simulink model "GD_Termoeletrica_Isolada_Droop"  (R2025b)
settings: Solver=ode23t  StartTime=0.0  StopTime=10  RelTol=1e-3  EnableMultiTasking=on
undefined symbols (not defined in the file): Three_PhaseV_IMeasuremen_class
libraries: fl_lib x9, nesl_utility x9, ee_lib x6, slpidlib x2, sdl_lib x2, AvgModels x1
settings Model: Creator=lgalo
settings SolverCC: AlgebraicLoopSolver=TrustRegion
settings DataIOCC: LimitDataPoints=on  SaveFormat=Array  ReturnWorkspaceOutputs=off
settings OptimizationCC: LifeSpan=inf
settings DebuggingCC: SaveWithParameterizedLinksMsg=none  UnconnectedInputMsg=warning  UnconnectedOutputMsg=warning  UnconnectedLineMsg=warning  SFUnexpectedBacktrackingDiag=warning  SFNoUnconditionalDefaultTransitionDiag=warning  SFExecutionAtInitializationDiag=none  ArithmeticOperatorsInVariantConditions=warning
settings HardwareCC: ProdBitPerPointer=32.0  ProdBitPerSizeT=32.0  ProdBitPerPtrDiffT=32.0  ProdLargestAtomicFloat=None  ProdIntDivRoundTo=Undefined  ProdEndianess=Unspecified  ProdWordSize=32.0  ProdHWDeviceType=32-bit Generic
settings ModelReferenceCC: PropagateSignalLabelsOutOfModel=off
settings SFSimCC: SimUseLocalCustomCode=off  CustomCodeUndefinedFunction=UseInterfaceOnly
settings RTWCC: RTWUseLocalCustomCode=off  GPUComputeCapability=3.5
settings CodeAppCC: StateflowObjectComments=on
settings GRTTargetCC: TargetLangStandard=C89/C90 (ANSI)
settings ConfigComp: CovMetricSettings=dw  CovSaveCumulativeToWorkspaceVar=on  CovSaveSingleToWorkspaceVar=on  CovExternalEMLEnable=off
settings SimscapeCC: SimscapeNormalizeSystem=off

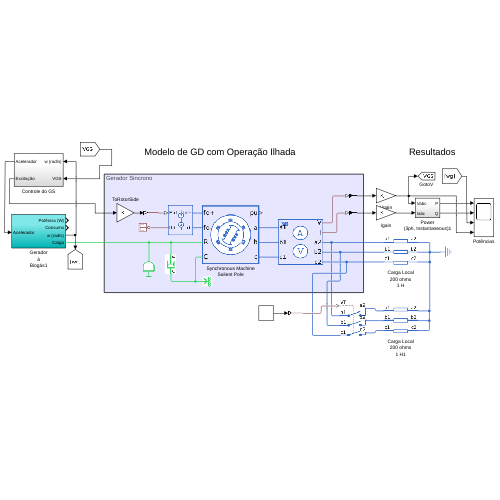
[thumbnail: Simulink's stored preview of the top-level diagram]
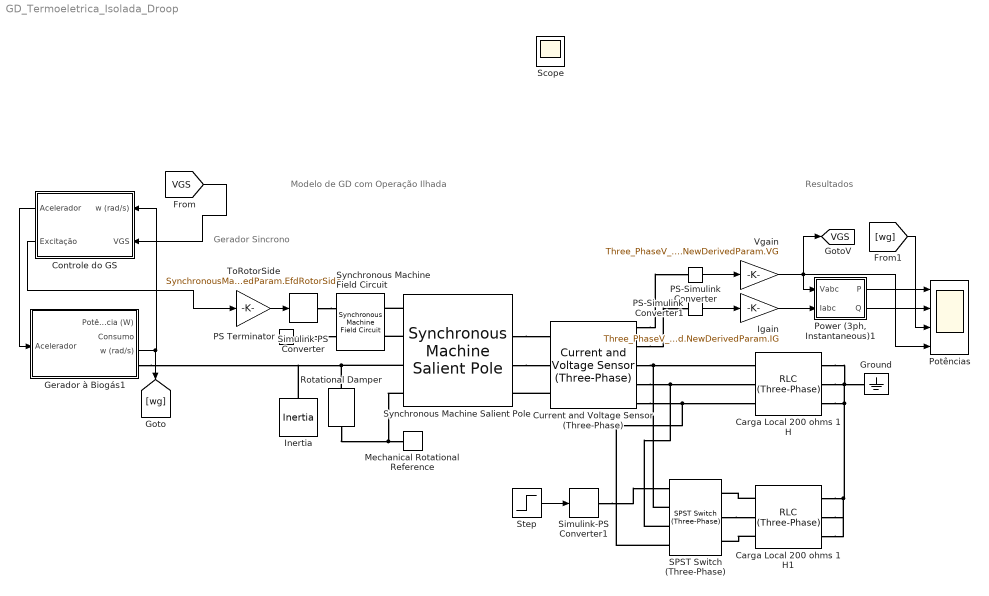
== system GD_Termoeletrica_Isolada_Droop ==
  note: Gerador Sincrono
  note: Modelo de GD com Operação Ilhada
  note: Resultados
  Carga Local 200 ohms 1 H : ee_lib/Passive/RLC Assemblies/RLC (Three-Phase)  port_option=ee.enum.threePhasePort.expanded  component_structure=8  R=200 Ohm  L=1 H  C=1e-06 F  R_parasitic=1e-6 Ohm  G_parasitic=1e-6 1/Ohm  IL_specify=on  IL_priority=High  IL=[0, 0, 0] A  IL_nominal_specify=off  IL_nominal_value=1  IL_nominal_unit=A  VC_specify=on  VC_priority=High  VC=[0, 0, 0] V  VC_nominal_specify=off  VC_nominal_value=1  VC_nominal_unit=V
      settings: InternalSimscapePortConfiguration="{\"Bottom\":[],\"Left\":[{\"id\":\"a1\",\"label\":\"a1\",\"type\":\"foundation.electrical.electrical\"},{\"id\":\"b1\",\"label\":\"b1\",\"type\":\"foundation.electrical.electrical\"},{\"id\":\"c1\",\"label\":\"c1\",\"type\":\"foundation.electrical.electrical\"}],\"Right\":[{\"id\":\"a2\",\"label\":\"a2\",\"type\":\"foundation.electrical.electrical\"},{\"id\":\"b2\",\"label\":\"b2\",\"type\":\"foundation.electrical.electrical\"},{\"id\":\"c2\",\"label\":\"c2\",\"type\":\"foundation.electrical.electrical\"}],\"Top\":[]}"
  Carga Local 200 ohms 1 H1 : ee_lib/Passive/RLC Assemblies/RLC (Three-Phase)  port_option=ee.enum.threePhasePort.expanded  component_structure=8  R=200 Ohm  L=1 H  C=1e-06 F  R_parasitic=1e-6 Ohm  G_parasitic=1e-6 1/Ohm  IL_specify=on  IL_priority=High  IL=[0, 0, 0] A  IL_nominal_specify=off  IL_nominal_value=1  IL_nominal_unit=A  VC_specify=on  VC_priority=High  VC=[0, 0, 0] V  VC_nominal_specify=off  VC_nominal_value=1  VC_nominal_unit=V
      settings: InternalSimscapePortConfiguration="{\"Bottom\":[],\"Left\":[{\"id\":\"a1\",\"label\":\"a1\",\"type\":\"foundation.electrical.electrical\"},{\"id\":\"b1\",\"label\":\"b1\",\"type\":\"foundation.electrical.electrical\"},{\"id\":\"c1\",\"label\":\"c1\",\"type\":\"foundation.electrical.electrical\"}],\"Right\":[{\"id\":\"a2\",\"label\":\"a2\",\"type\":\"foundation.electrical.electrical\"},{\"id\":\"b2\",\"label\":\"b2\",\"type\":\"foundation.electrical.electrical\"},{\"id\":\"c2\",\"label\":\"c2\",\"type\":\"foundation.electrical.electrical\"}],\"Top\":[]}"
  Controle do GS : Subsystem
  Current and Voltage Sensor (Three-Phase) : ee_lib/Sensors & Transducers/Current and Voltage Sensor (Three-Phase)  vMeasurementType=2  outputUnit=2  SRated=100000000 V*A  VRated=500000 V  I_specify=off  I_priority=None  I=[ 0 0 0 ] A  I_nominal_specify=off  I_nominal_value=1  I_nominal_unit=A  V_specify=off  V_priority=None  V=[ 0 0 0 ] V  V_nominal_specify=off  V_nominal_value=1  V_nominal_unit=V
      settings: InternalSimscapePortConfiguration="{\"Bottom\":[],\"Left\":[{\"id\":\"a1\",\"label\":\"a1\",\"type\":\"foundation.electrical.electrical\"},{\"id\":\"b1\",\"label\":\"b1\",\"type\":\"foundation.electrical.electrical\"},{\"id\":\"c1\",\"label\":\"c1\",\"type\":\"foundation.electrical.electrical\"}],\"Right\":[{\"id\":\"V_output\",\"label\":\"V\",\"type\":\"output\"},{\"id\":\"I_output\",\"label\":\"I\",\"type\":\"output\"},{\"id\":\"a2\",\"label\":\"a2\",\"type\":\"foundation.electrical.electrical\"},{\"id\":\"b2\",\"label\":\"b2\",\"type\":\"foundation.electrical.electrical\"},{\"id\":\"c2\",\"label\":\"c2\",\"type\":\"foundation.electrical.electrical\"}],\"Top\":[]}"
  Gerador à Biogás1 : Subsystem
  Ground : fl_lib/Electrical/Electrical Elements/Electrical Reference
  Igain : Gain  Gain=Three_PhaseV_IMeasuremen_class('phase-to-ground','yes','off','off','off',100000000,500000).objParamMappingDerived.NewDerivedParam.IG
  Inertia : fl_lib/Mechanical/Rotational Elements/Inertia  inertia=SynchronousMachineSIFund_class('Mechanical rotational port',[20000 460 60],[0.645 0.002217 0.05296 0.0252],[0.1279 0.016 2],2,[0 0 0 0 0 0 0 0 1.3192],[695.64 774.7 917.5 1001.6 1082.2 1175.9 1293.6 1430.2 1583.7;9660 10623 12243 13063 13757 14437 15180 15890 16567],'off',[0.0664 0.001387 0.0292 0.0006896 0.007907 0.002477],[1.137 0.00419 1.54 0.004893],[0.3802 0.005517],'Salient-pole').objParamMappingDerived.NewDerivedParam.J kg*m^2  num_ports=foundation.enum.numPorts2.one  w_specify=on  w_priority=Low  w=SynchronousMachineSIFund_class('Mechanical rotational port',[20000 460 60],[0.645 0.002217 0.05296 0.0252],[0.1279 0.016 2],2,[0 0 0 0 0 0 0 0 1.3192],[695.64 774.7 917.5 1001.6 1082.2 1175.9 1293.6 1430.2 1583.7;9660 10623 12243 13063 13757 14437 15180 15890 16567],'off',[0.0664 0.001387 0.0292 0.0006896 0.007907 0.002477],[1.137 0.00419 1.54 0.004893],[0.3802 0.005517],'Salient-pole').objParamMappingDerived.NewDerivedParam.wrm0 rad/s  w_nominal_specify=off  w_nominal_value=1  w_nominal_unit=rad/s  t_specify=off  t_priority=None  t=0 N*m  t_nominal_specify=off  t_nominal_value=1  t_nominal_unit=N*m
  Mechanical Rotational Reference : fl_lib/Mechanical/Rotational Elements/Mechanical Rotational Reference
  PS Terminator : fl_lib/Physical Signals/Sinks/PS Terminator
  PS-Simulink Converter : nesl_utility/PS-Simulink Converter  PhysicalDomain=network_engine_domain  SubClassName=ps_output  LeftPortType=input  RightPortType=output  PseudoPeriodic=off  Frequencies=[]  VectorFormat=1-D array  Unit=1  AffineConversion=off
  PS-Simulink Converter1 : nesl_utility/PS-Simulink Converter  PhysicalDomain=network_engine_domain  SubClassName=ps_output  LeftPortType=input  RightPortType=output  PseudoPeriodic=off  Frequencies=[]  VectorFormat=1-D array  Unit=1  AffineConversion=off
  Potências : Scope  NumInputPorts=4
      settings: TimeSpan=10  ActiveDisplayYMinimum=-98.69848861877999  ActiveDisplayYMaximum=888.28639756902021  DataLoggingSaveFormat=Array
  "Power (3ph, Instantaneous)1" : Subsystem
  Rotational Damper : fl_lib/Mechanical/Rotational Elements/Rotational Damper  D=SynchronousMachineSIFund_class('Mechanical rotational port',[20000 460 60],[0.645 0.002217 0.05296 0.0252],[0.1279 0.016 2],2,[0 0 0 0 0 0 0 0 1.3192],[695.64 774.7 917.5 1001.6 1082.2 1175.9 1293.6 1430.2 1583.7;9660 10623 12243 13063 13757 14437 15180 15890 16567],'off',[0.0664 0.001387 0.0292 0.0006896 0.007907 0.002477],[1.137 0.00419 1.54 0.004893],[0.3802 0.005517],'Salient-pole').objParamMappingDerived.NewDerivedParam.D N*m/(rad/s)  w_specify=on  w_priority=Low  w=SynchronousMachineSIFund_class('Mechanical rotational port',[20000 460 60],[0.645 0.002217 0.05296 0.0252],[0.1279 0.016 2],2,[0 0 0 0 0 0 0 0 1.3192],[695.64 774.7 917.5 1001.6 1082.2 1175.9 1293.6 1430.2 1583.7;9660 10623 12243 13063 13757 14437 15180 15890 16567],'off',[0.0664 0.001387 0.0292 0.0006896 0.007907 0.002477],[1.137 0.00419 1.54 0.004893],[0.3802 0.005517],'Salient-pole').objParamMappingDerived.NewDerivedParam.wrm0 rad/s  w_nominal_specify=off  w_nominal_value=1  w_nominal_unit=rad/s  t_specify=off  t_priority=None  t=0 N*m  t_nominal_specify=off  t_nominal_value=1  t_nominal_unit=N*m
  SPST Switch (Three-Phase) : ee_lib/Switches & Breakers/SPST Switch (Three-Phase)  R_closed=0.001 Ohm  G_open=1e-6 1/Ohm  threshold=0.5 V  i_vT_specify=off  i_vT_priority=None  i_vT=0 A  i_vT_nominal_specify=off  i_vT_nominal_value=1  i_vT_nominal_unit=A  I_specify=off  I_priority=None  I=[0, 0, 0] A  I_nominal_specify=off  I_nominal_value=1  I_nominal_unit=A  V_specify=off  V_priority=None  V=[0, 0, 0] V  V_nominal_specify=off  V_nominal_value=1  V_nominal_unit=V  i_a_specify=off  i_a_priority=None  i_a=0 A  i_a_nominal_specify=off  i_a_nominal_value=1  i_a_nominal_unit=A  v_a_specify=off  v_a_priority=None  v_a=0 V  v_a_nominal_specify=off  v_a_nominal_value=1  v_a_nominal_unit=V  i_b_specify=off  i_b_priority=None  i_b=0 A  i_b_nominal_specify=off  i_b_nominal_value=1  i_b_nominal_unit=A  v_b_specify=off  v_b_priority=None  v_b=0 V  v_b_nominal_specify=off  v_b_nominal_value=1  v_b_nominal_unit=V  i_c_specify=off  i_c_priority=None  i_c=0 A  i_c_nominal_specify=off  i_c_nominal_value=1  i_c_nominal_unit=A  v_c_specify=off  v_c_priority=None  v_c=0 V  v_c_nominal_specify=off  v_c_nominal_value=1  v_c_nominal_unit=V
      settings: InternalSimscapePortConfiguration="{\"Bottom\":[],\"Left\":[{\"id\":\"vT\",\"label\":\"vT\",\"type\":\"input\"},{\"id\":\"a1\",\"label\":\"a1\",\"type\":\"foundation.electrical.electrical\"},{\"id\":\"b1\",\"label\":\"b1\",\"type\":\"foundation.electrical.electrical\"},{\"id\":\"c1\",\"label\":\"c1\",\"type\":\"foundation.electrical.electrical\"}],\"Right\":[{\"id\":\"a2\",\"label\":\"a2\",\"type\":\"foundation.electrical.electrical\"},{\"id\":\"b2\",\"label\":\"b2\",\"type\":\"foundation.electrical.electrical\"},{\"id\":\"c2\",\"label\":\"c2\",\"type\":\"foundation.electrical.electrical\"}],\"Top\":[]}"
  Simulink-PS Converter : nesl_utility/Simulink-PS Converter  PhysicalDomain=network_engine_domain  SubClassName=ps_input  LeftPortType=input  RightPortType=output  PseudoPeriodic=off  Frequencies=[]  NoiseDistribution=none  NoiseParameters=[]  Unit=1  AffineConversion=off  FilteringAndDerivatives=provide  SimscapeFilterOrder=1  InputFilterTimeConstant=0.001  UdotUserProvided=0
  Simulink-PS Converter1 : nesl_utility/Simulink-PS Converter  PhysicalDomain=network_engine_domain  SubClassName=ps_input  LeftPortType=input  RightPortType=output  PseudoPeriodic=off  Frequencies=[]  NoiseDistribution=none  NoiseParameters=[]  Unit=1  AffineConversion=off  FilteringAndDerivatives=provide  SimscapeFilterOrder=1  InputFilterTimeConstant=0.001  UdotUserProvided=0
  Step : Step  Time=5  SampleTime=0
  Synchronous Machine Field Circuit : ee_lib/Electromechanical/Synchronous/Synchronous Machine Field Circuit  unit_option=ee.enum.unit.si  SRated=555e6 V*A  FRated=60 Hz  fieldCircuitParameterization_option=ee.enum.sm.fieldparameterization.current  baseEfd=92.95 V  baseIfd=1300 A  parameterization_option=ee.enum.sm.parameterization.fundamental  Ladu=1.66  Rfd=0.0006  Xl=0.15  Xd=1.81  Xdd=0.3  Xddd=0.23  d_option=ee.enum.circuit.open  Td0d=8 s  Tdd=1.3260 s  Td0dd=0.03 s  Tddd=0.0230 s
      settings: InternalSimscapePortConfiguration="{\"Bottom\":[],\"Left\":[{\"id\":\"Efd\",\"label\":\"Efd\",\"type\":\"input\"},{\"id\":\"Ifd\",\"label\":\"Ifd\",\"type\":\"output\"}],\"Right\":[{\"id\":\"fd_p\",\"label\":\"fd+\",\"type\":\"foundation.electrical.electrical\"},{\"id\":\"fd_n\",\"label\":\"fd-\",\"type\":\"foundation.electrical.electrical\"}],\"Top\":[]}"
  Synchronous Machine Salient Pole : ee_lib/Electromechanical/Synchronous/Synchronous Machine Salient Pole  port_option=ee.enum.threePhasePort.expanded  SRated=SynchronousMachineSIFund_class('Mechanical rotational port',[20000 460 60],[0.645 0.002217 0.05296 0.0252],[0.1279 0.016 2],2,[0 0 0 0 0 0 0 0 1.3192],[695.64 774.7 917.5 1001.6 1082.2 1175.9 1293.6 1430.2 1583.7;9660 10623 12243 13063 13757 14437 15180 15890 16567],'off',[0.0664 0.001387 0.0292 0.0006896 0.007907 0.002477],[1.137 0.00419 1.54 0.004893],[0.3802 0.005517],'Salient-pole').objParamMappingDerived.NewDerivedParam.SRated V*A  VRated=SynchronousMachineSIFund_class('Mechanical rotational port',[20000 460 60],[0.645 0.002217 0.05296 0.0252],[0.1279 0.016 2],2,[0 0 0 0 0 0 0 0 1.3192],[695.64 774.7 917.5 1001.6 1082.2 1175.9 1293.6 1430.2 1583.7;9660 10623 12243 13063 13757 14437 15180 15890 16567],'off',[0.0664 0.001387 0.0292 0.0006896 0.007907 0.002477],[1.137 0.00419 1.54 0.004893],[0.3802 0.005517],'Salient-pole').objParamMappingDerived.NewDerivedParam.VRated V  FRated=SynchronousMachineSIFund_class('Mechanical rotational port',[20000 460 60],[0.645 0.002217 0.05296 0.0252],[0.1279 0.016 2],2,[0 0 0 0 0 0 0 0 1.3192],[695.64 774.7 917.5 1001.6 1082.2 1175.9 1293.6 1430.2 1583.7;9660 10623 12243 13063 13757 14437 15180 15890 16567],'off',[0.0664 0.001387 0.0292 0.0006896 0.007907 0.002477],[1.137 0.00419 1.54 0.004893],[0.3802 0.005517],'Salient-pole').objParamMappingDerived.NewDerivedParam.FRated Hz  nPolePairs=SynchronousMachineSIFund_class('Mechanical rotational port',[20000 460 60],[0.645 0.002217 0.05296 0.0252],[0.1279 0.016 2],2,[0 0 0 0 0 0 0 0 1.3192],[695.64 774.7 917.5 1001.6 1082.2 1175.9 1293.6 1430.2 1583.7;9660 10623 12243 13063 13757 14437 15180 15890 16567],'off',[0.0664 0.001387 0.0292 0.0006896 0.007907 0.002477],[1.137 0.00419 1.54 0.004893],[0.3802 0.005517],'Salient-pole').objParamMappingDerived.NewDerivedParam.nPolePairs  param_option=ee.enum.sm.parameterization.fundamental  fieldCircuitParameterization_option=ee.enum.sm.fieldparameterization.current  baseEfd=216.54 V  baseIfd=SynchronousMachineSIFund_class('Mechanical rotational port',[20000 460 60],[0.645 0.002217 0.05296 0.0252],[0.1279 0.016 2],2,[0 0 0 0 0 0 0 0 1.3192],[695.64 774.7 917.5 1001.6 1082.2 1175.9 1293.6 1430.2 1583.7;9660 10623 12243 13063 13757 14437 15180 15890 16567],'off',[0.0664 0.001387 0.0292 0.0006896 0.007907 0.002477],[1.137 0.00419 1.54 0.004893],[0.3802 0.005517],'Salient-pole').objParamMappingDerived.NewDerivedParam.baseIfd A  zero_sequence=ee.enum.park.zerosequence.exclude  axes_param=ee.enum.rotorangle.qaxis  Ladu=SynchronousMachineSIFund_class('Mechanical rotational port',[20000 460 60],[0.645 0.002217 0.05296 0.0252],[0.1279 0.016 2],2,[0 0 0 0 0 0 0 0 1.3192],[695.64 774.7 917.5 1001.6 1082.2 1175.9 1293.6 1430.2 1583.7;9660 10623 12243 13063 13757 14437 15180 15890 16567],'off',[0.0664 0.001387 0.0292 0.0006896 0.007907 0.002477],[1.137 0.00419 1.54 0.004893],[0.3802 0.005517],'Salient-pole').objParamMappingDerived.NewDerivedParam.Ladu  Laqu=SynchronousMachineSIFund_class('Mechanical rotational port',[20000 460 60],[0.645 0.002217 0.05296 0.0252],[0.1279 0.016 2],2,[0 0 0 0 0 0 0 0 1.3192],[695.64 774.7 917.5 1001.6 1082.2 1175.9 1293.6 1430.2 1583.7;9660 10623 12243 13063 13757 14437 15180 15890 16567],'off',[0.0664 0.001387 0.0292 0.0006896 0.007907 0.002477],[1.137 0.00419 1.54 0.004893],[0.3802 0.005517],'Salient-pole').objParamMappingDerived.NewDerivedParam.Laqu  L0=SynchronousMachineSIFund_class('Mechanical rotational port',[20000 460 60],[0.645 0.002217 0.05296 0.0252],[0.1279 0.016 2],2,[0 0 0 0 0 0 0 0 1.3192],[695.64 774.7 917.5 1001.6 1082.2 1175.9 1293.6 1430.2 1583.7;9660 10623 12243 13063 13757 14437 15180 15890 16567],'off',[0.0664 0.001387 0.0292 0.0006896 0.007907 0.002477],[1.137 0.00419 1.54 0.004893],[0.3802 0.005517],'Salient-pole').objParamMappingDerived.NewDerivedParam.L0  Ll=SynchronousMachineSIFund_class('Mechanical rotational port',[20000 460 60],[0.645 0.002217 0.05296 0.0252],[0.1279 0.016 2],2,[0 0 0 0 0 0 0 0 1.3192],[695.64 774.7 917.5 1001.6 1082.2 1175.9 1293.6 1430.2 1583.7;9660 10623 12243 13063 13757 14437 15180 15890 16567],'off',[0.0664 0.001387 0.0292 0.0006896 0.007907 0.002477],[1.137 0.00419 1.54 0.004893],[0.3802 0.005517],'Salient-pole').objParamMappingDerived.NewDerivedParam.Ll  Ra=SynchronousMachineSIFund_class('Mechanical rotational port',[20000 460 60],[0.645 0.002217 0.05296 0.0252],[0.1279 0.016 2],2,[0 0 0 0 0 0 0 0 1.3192],[695.64 774.7 917.5 1001.6 1082.2 1175.9 1293.6 1430.2 1583.7;9660 10623 12243 13063 13757 14437 15180 15890 16567],'off',[0.0664 0.001387 0.0292 0.0006896 0.007907 0.002477],[1.137 0.00419 1.54 0.004893],[0.3802 0.005517],'Salient-pole').objParamMappingDerived.NewDerivedParam.Ra  Lfd=SynchronousMachineSIFund_class('Mechanical rotational port',[20000 460 60],[0.645 0.002217 0.05296 0.0252],[0.1279 0.016 2],2,[0 0 0 0 0 0 0 0 1.3192],[695.64 774.7 917.5 1001.6 1082.2 1175.9 1293.6 1430.2 1583.7;9660 10623 12243 13063 13757 14437 15180 15890 16567],'off',[0.0664 0.001387 0.0292 0.0006896 0.007907 0.002477],[1.137 0.00419 1.54 0.004893],[0.3802 0.005517],'Salient-pole').objParamMappingDerived.NewDerivedParam.Lfd  Rfd=SynchronousMachineSIFund_class('Mechanical rotational port',[20000 460 60],[0.645 0.002217 0.05296 0.0252],[0.1279 0.016 2],2,[0 0 0 0 0 0 0 0 1.3192],[695.64 774.7 917.5 1001.6 1082.2 1175.9 1293.6 1430.2 1583.7;9660 10623 12243 13063 13757 14437 15180 15890 16567],'off',[0.0664 0.001387 0.0292 0.0006896 0.007907 0.002477],[1.137 0.00419 1.54 0.004893],[0.3802 0.005517],'Salient-pole').objParamMappingDerived.NewDerivedParam.Rfd  L1d=SynchronousMachineSIFund_class('Mechanical rotational port',[20000 460 60],[0.645 0.002217 0.05296 0.0252],[0.1279 0.016 2],2,[0 0 0 0 0 0 0 0 1.3192],[695.64 774.7 917.5 1001.6 1082.2 1175.9 1293.6 1430.2 1583.7;9660 10623 12243 13063 13757 14437 15180 15890 16567],'off',[0.0664 0.001387 0.0292 0.0006896 0.007907 0.002477],[1.137 0.00419 1.54 0.004893],[0.3802 0.005517],'Salient-pole').objParamMappingDerived.NewDerivedParam.L1d  R1d=SynchronousMachineSIFund_class('Mechanical rotational port',[20000 460 60],[0.645 0.002217 0.05296 0.0252],[0.1279 0.016 2],2,[0 0 0 0 0 0 0 0 1.3192],[695.64 774.7 917.5 1001.6 1082.2 1175.9 1293.6 1430.2 1583.7;9660 10623 12243 13063 13757 14437 15180 15890 16567],'off',[0.0664 0.001387 0.0292 0.0006896 0.007907 0.002477],[1.137 0.00419 1.54 0.004893],[0.3802 0.005517],'Salient-pole').objParamMappingDerived.NewDerivedParam.R1d  L1q=SynchronousMachineSIFund_class('Mechanical rotational port',[20000 460 60],[0.645 0.002217 0.05296 0.0252],[0.1279 0.016 2],2,[0 0 0 0 0 0 0 0 1.3192],[695.64 774.7 917.5 1001.6 1082.2 1175.9 1293.6 1430.2 1583.7;9660 10623 12243 13063 13757 14437 15180 15890 16567],'off',[0.0664 0.001387 0.0292 0.0006896 0.007907 0.002477],[1.137 0.00419 1.54 0.004893],[0.3802 0.005517],'Salient-pole').objParamMappingDerived.NewDerivedParam.L1q  R1q=SynchronousMachineSIFund_class('Mechanical rotational port',[20000 460 60],[0.645 0.002217 0.05296 0.0252],[0.1279 0.016 2],2,[0 0 0 0 0 0 0 0 1.3192],[695.64 774.7 917.5 1001.6 1082.2 1175.9 1293.6 1430.2 1583.7;9660 10623 12243 13063 13757 14437 15180 15890 16567],'off',[0.0664 0.001387 0.0292 0.0006896 0.007907 0.002477],[1.137 0.00419 1.54 0.004893],[0.3802 0.005517],'Salient-pole').objParamMappingDerived.NewDerivedParam.R1q  Xl=0.15  Xd=1.05  Xq=0.7  X0=0.15  Xdd=0.35  Xddd=0.25  Xqdd=0.325  d_option=ee.enum.circuit.open  Td0d=5.25 s  Tdd=1.75 s  Td0dd=0.03 s  Tddd=0.0214 s  q_option=ee.enum.circuit.open  Tq0dd=0.05 s  Tqdd=0.0232 s  saturation_option=0  saturation_ifd=SynchronousMachineSIFund_class('Mechanical rotational port',[20000 460 60],[0.645 0.002217 0.05296 0.0252],[0.1279 0.016 2],2,[0 0 0 0 0 0 0 0 1.3192],[695.64 774.7 917.5 1001.6 1082.2 1175.9 1293.6 1430.2 1583.7;9660 10623 12243 13063 13757 14437 15180 15890 16567],'off',[0.0664 0.001387 0.0292 0.0006896 0.007907 0.002477],[1.137 0.00419 1.54 0.004893],[0.3802 0.005517],'Salient-pole').objParamMappingDerived.NewDerivedParam.saturation_ifd  saturation_Vag=SynchronousMachineSIFund_class('Mechanical rotational port',[20000 460 60],[0.645 0.002217 0.05296 0.0252],[0.1279 0.016 2],2,[0 0 0 0 0 0 0 0 1.3192],[695.64 774.7 917.5 1001.6 1082.2 1175.9 1293.6 1430.2 1583.7;9660 10623 12243 13063 13757 14437 15180 15890 16567],'off',[0.0664 0.001387 0.0292 0.0006896 0.007907 0.002477],[1.137 0.00419 1.54 0.004893],[0.3802 0.005517],'Salient-pole').objParamMappingDerived.NewDerivedParam.saturation_Vag  initialization_option=ee.enum.sm.initialization.mechanical  source_type=ee.enum.sm.load_flow_source_type.Swing  Vmag0=24e3 V  Vang0=0 deg  Pt0=270e6 V*A  Qt0=0 V*A  minimum_pu=0.95  phase_search_range=[-30, 30] deg  gmin=1e-6 S  connection_option=ee.enum.Connection.wye  num_q_dampers=1  rotor_offset=-pi / 2 rad  pu_psid_specify=on  pu_psid_priority=High  pu_psid=SynchronousMachineSIFund_class('Mechanical rotational port',[20000 460 60],[0.645 0.002217 0.05296 0.0252],[0.1279 0.016 2],2,[0 0 0 0 0 0 0 0 1.3192],[695.64 774.7 917.5 1001.6 1082.2 1175.9 1293.6 1430.2 1583.7;9660 10623 12243 13063 13757 14437 15180 15890 16567],'off',[0.0664 0.001387 0.0292 0.0006896 0.007907 0.002477],[1.137 0.00419 1.54 0.004893],[0.3802 0.005517],'Salient-pole').objParamMappingDerived.NewDerivedParam.pu_psid0  pu_psid_nominal_specify=off  pu_psid_nominal_value=1  pu_psid_nominal_unit=1  pu_psiq_specify=on  pu_psiq_priority=High  pu_psiq=SynchronousMachineSIFund_class('Mechanical rotational port',[20000 460 60],[0.645 0.002217 0.05296 0.0252],[0.1279 0.016 2],2,[0 0 0 0 0 0 0 0 1.3192],[695.64 774.7 917.5 1001.6 1082.2 1175.9 1293.6 1430.2 1583.7;9660 10623 12243 13063 13757 14437 15180 15890 16567],'off',[0.0664 0.001387 0.0292 0.0006896 0.007907 0.002477],[1.137 0.00419 1.54 0.004893],[0.3802 0.005517],'Salient-pole').objParamMappingDerived.NewDerivedParam.pu_psiq0  pu_psiq_nominal_specify=off  pu_psiq_nominal_value=1  pu_psiq_nominal_unit=1  pu_psifd_specify=on  pu_psifd_priority=High  pu_psifd=SynchronousMachineSIFund_class('Mechanical rotational port',[20000 460 60],[0.645 0.002217 0.05296 0.0252],[0.1279 0.016 2],2,[0 0 0 0 0 0 0 0 1.3192],[695.64 774.7 917.5 1001.6 1082.2 1175.9 1293.6 1430.2 1583.7;9660 10623 12243 13063 13757 14437 15180 15890 16567],'off',[0.0664 0.001387 0.0292 0.0006896 0.007907 0.002477],[1.137 0.00419 1.54 0.004893],[0.3802 0.005517],'Salient-pole').objParamMappingDerived.NewDerivedParam.pu_psifd0  pu_psifd_nominal_specify=off  pu_psifd_nominal_value=1  pu_psifd_nominal_unit=1  pu_psi1d_specify=on  pu_psi1d_priority=High  pu_psi1d=SynchronousMachineSIFund_class('Mechanical rotational port',[20000 460 60],[0.645 0.002217 0.05296 0.0252],[0.1279 0.016 2],2,[0 0 0 0 0 0 0 0 1.3192],[695.64 774.7 917.5 1001.6 1082.2 1175.9 1293.6 1430.2 1583.7;9660 10623 12243 13063 13757 14437 15180 15890 16567],'off',[0.0664 0.001387 0.0292 0.0006896 0.007907 0.002477],[1.137 0.00419 1.54 0.004893],[0.3802 0.005517],'Salient-pole').objParamMappingDerived.NewDerivedParam.pu_psi1d0  pu_psi1d_nominal_specify=off  pu_psi1d_nominal_value=1  pu_psi1d_nominal_unit=1  pu_psi1q_specify=on  pu_psi1q_priority=High  pu_psi1q=SynchronousMachineSIFund_class('Mechanical rotational port',[20000 460 60],[0.645 0.002217 0.05296 0.0252],[0.1279 0.016 2],2,[0 0 0 0 0 0 0 0 1.3192],[695.64 774.7 917.5 1001.6 1082.2 1175.9 1293.6 1430.2 1583.7;9660 10623 12243 13063 13757 14437 15180 15890 16567],'off',[0.0664 0.001387 0.0292 0.0006896 0.007907 0.002477],[1.137 0.00419 1.54 0.004893],[0.3802 0.005517],'Salient-pole').objParamMappingDerived.NewDerivedParam.pu_psi1q0  pu_psi1q_nominal_specify=off  pu_psi1q_nominal_value=1  pu_psi1q_nominal_unit=1  angular_position_diff_specify=on  angular_position_diff_priority=High  angular_position_diff=SynchronousMachineSIFund_class('Mechanical rotational port',[20000 460 60],[0.645 0.002217 0.05296 0.0252],[0.1279 0.016 2],2,[0 0 0 0 0 0 0 0 1.3192],[695.64 774.7 917.5 1001.6 1082.2 1175.9 1293.6 1430.2 1583.7;9660 10623 12243 13063 13757 14437 15180 15890 16567],'off',[0.0664 0.001387 0.0292 0.0006896 0.007907 0.002477],[1.137 0.00419 1.54 0.004893],[0.3802 0.005517],'Salient-pole').objParamMappingDerived.NewDerivedParam.thm0 deg  angular_position_diff_nominal_specify=off  angular_position_diff_nominal_value=1  angular_position_diff_nominal_unit=deg  Tmeas=298.15 K  alpha=3.93e-3 1/K  stator_thermal_mass=100 J/K  rotor_thermal_mass=200 J/K  temperatureA_specify=off  temperatureA_priority=High  temperatureA=25 degC  temperatureA_nominal_specify=off  temperatureA_nominal_value=1  temperatureA_nominal_unit=degC  temperatureB_specify=off  temperatureB_priority=High  temperatureB=25 degC  temperatureB_nominal_specify=off  temperatureB_nominal_value=1  temperatureB_nominal_unit=degC  temperatureC_specify=off  temperatureC_priority=High  temperatureC=25 degC  temperatureC_nominal_specify=off  temperatureC_nominal_value=1  temperatureC_nominal_unit=degC  temperatureR_specify=off  temperatureR_priority=High  temperatureR=25 degC  temperatureR_nominal_specify=off  temperatureR_nominal_value=1  temperatureR_nominal_unit=degC
      settings: InternalSimscapePortConfiguration="{\"Bottom\":[],\"Left\":[{\"id\":\"fd_p\",\"label\":\"fd+\",\"type\":\"foundation.electrical.electrical\"},{\"id\":\"fd_n\",\"label\":\"fd-\",\"type\":\"foundation.electrical.electrical\"},{\"id\":\"R\",\"label\":\"R\",\"type\":\"foundation.mechanical.rotational.rotational\"},{\"id\":\"C\",\"label\":\"C\",\"type\":\"foundation.mechanical.rotational.rotational\"}],\"Right\":[{\"id\":\"pu_output\",\"label\":\"pu\",\"type\":\"output\"},{\"id\":\"a\",\"label\":\"a\",\"type\":\"foundation.electrical.electrical\"},{\"id\":\"b\",\"label\":\"b\",\"type\":\"foundation.electrical.electrical\"},{\"id\":\"c\",\"label\":\"c\",\"type\":\"foundation.electrical.electrical\"}],\"Top\":[]}"
  ToRotorSide : Gain  Gain=SynchronousMachineSIFund_class('Mechanical rotational port',[20000 460 60],[0.645 0.002217 0.05296 0.0252],[0.1279 0.016 2],2,[0 0 0 0 0 0 0 0 1.3192],[695.64 774.7 917.5 1001.6 1082.2 1175.9 1293.6 1430.2 1583.7;9660 10623 12243 13063 13757 14437 15180 15890 16567],'off',[0.0664 0.001387 0.0292 0.0006896 0.007907 0.002477],[1.137 0.00419 1.54 0.004893],[0.3802 0.005517],'Salient-pole').objParamMappingDerived.NewDerivedParam.EfdRotorSide
  Vgain : Gain  Gain=Three_PhaseV_IMeasuremen_class('phase-to-ground','yes','off','off','off',100000000,500000).objParamMappingDerived.NewDerivedParam.VG
  Scope : Scope
      settings: ActiveDisplayYMinimum=-7.7846435147940412  ActiveDisplayYMaximum=70.061791633146385
  tag scope: VGS=global
  wires:
  Gerador à Biogás1/3(w (rad/s)) -> Controle do GS/1(w (rad/s)), [wg]
  Igain/1 -> "Power (3ph, Instantaneous)1"/2(Iabc)
  Vgain/1 -> [VGS], "Power (3ph, Instantaneous)1"/1(Vabc), Potências/4
  "Power (3ph, Instantaneous)1"/1(P) -> Potências/1
  "Power (3ph, Instantaneous)1"/2(Q) -> Potências/2
  Controle do GS/2(Excitação) -> ToRotorSide/1
  ToRotorSide/1 -> Simulink-PS Converter/1
  PS-Simulink Converter1/1 -> Igain/1
  PS-Simulink Converter/1 -> Vgain/1
  Controle do GS/1(Acelerador) -> Gerador à Biogás1/1(Acelerador)
  [VGS] -> Controle do GS/2(VGS)
  [wg] -> Potências/3
  Step/1 -> Simulink-PS Converter1/1
  connections:
  Carga Local 200 ohms 1 H1/RConn1 -- Ground/LConn1 -- Carga Local 200 ohms 1 H/RConn1 -- Carga Local 200 ohms 1 H/RConn2 -- Carga Local 200 ohms 1 H/RConn3 -- Carga Local 200 ohms 1 H1/RConn3 -- Carga Local 200 ohms 1 H1/RConn2
  Synchronous Machine Salient Pole/LConn3 -- Gerador à Biogás1/RConn1 -- Inertia/LConn1 -- Rotational Damper/LConn1
  Rotational Damper/RConn1 -- Synchronous Machine Salient Pole/LConn4 -- Mechanical Rotational Reference/LConn1
  Synchronous Machine Salient Pole/RConn2 -- Current and Voltage Sensor (Three-Phase)/LConn1
  Synchronous Machine Salient Pole/LConn1 -- Synchronous Machine Field Circuit/RConn1
  Synchronous Machine Salient Pole/LConn2 -- Synchronous Machine Field Circuit/RConn2
  Current and Voltage Sensor (Three-Phase)/LConn3 -- Synchronous Machine Salient Pole/RConn4
  Synchronous Machine Salient Pole/RConn3 -- Current and Voltage Sensor (Three-Phase)/LConn2
  Simulink-PS Converter/RConn1 -- Synchronous Machine Field Circuit/LConn1
  PS Terminator/LConn1 -- Synchronous Machine Field Circuit/LConn2
  Current and Voltage Sensor (Three-Phase)/RConn1 -- PS-Simulink Converter/LConn1
  Current and Voltage Sensor (Three-Phase)/RConn2 -- PS-Simulink Converter1/LConn1
  Current and Voltage Sensor (Three-Phase)/RConn3 -- Carga Local 200 ohms 1 H/LConn1 -- SPST Switch (Three-Phase)/LConn2
  Current and Voltage Sensor (Three-Phase)/RConn4 -- SPST Switch (Three-Phase)/LConn3 -- Carga Local 200 ohms 1 H/LConn2
  Current and Voltage Sensor (Three-Phase)/RConn5 -- SPST Switch (Three-Phase)/LConn4 -- Carga Local 200 ohms 1 H/LConn3
  Carga Local 200 ohms 1 H1/LConn3 -- SPST Switch (Three-Phase)/RConn3
  Carga Local 200 ohms 1 H1/LConn1 -- SPST Switch (Three-Phase)/RConn1
  Simulink-PS Converter1/RConn1 -- SPST Switch (Three-Phase)/LConn1
  SPST Switch (Three-Phase)/RConn2 -- Carga Local 200 ohms 1 H1/LConn2

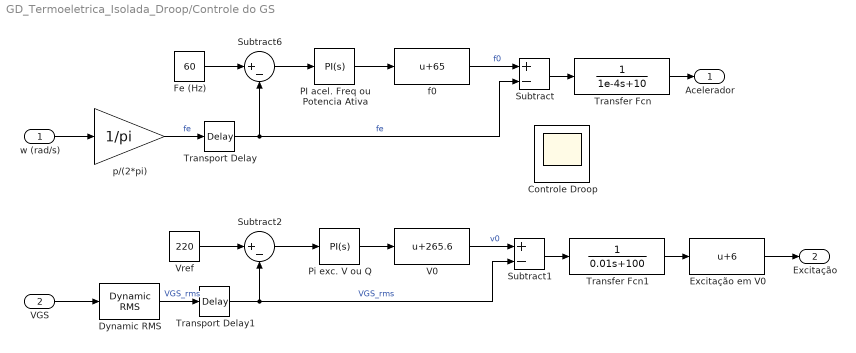
== system GD_Termoeletrica_Isolada_Droop/Controle do GS ==
  w (rad/s) : Inport
  VGS : Inport  Port=2
  Controle Droop : Scope
      settings: IsFloating=on  Floating=on  TimeSpan=10  ActiveDisplayYMinimum=35  ActiveDisplayYMaximum=95  DataLoggingMaxPoints=10000  DataLoggingVariableName=ScopeData3  DataLoggingSaveFormat=Array
  Dynamic RMS : AvgModels/Calculos/Dynamic RMS  nfases=3  fbase=60
      settings: SourceProductName=SimAverageModels
  Excitação em V0 : Bias  Bias=6  SaturateOnIntegerOverflow=off
  Fe (Hz) : Constant  Value=60
  PI acel. Freq ou Potencia Ativa : slpidlib/PID Controller  Controller=PI  Form=Parallel  TimeDomain=Continuous-time  UseExternalTs=off  SampleTime=-1  IntegratorMethod=Forward Euler  FilterMethod=Forward Euler  ControllerParametersSource=internal  P=1  I=5  UseKiTs=off  D=0  UseExternalDerivativeSource=off  N=100  UseFilter=on  TunerSelectOption=Transfer Function Based (PID Tuner App)  InitialConditionSource=internal  InitialConditionForIntegrator=0.5  InitialConditionForFilter=0  DifferentiatorICPrevScaledInput=0  ExternalReset=none  TrackingMode=off  Kt=1  LimitOutput=on  SatLimitsSource=internal  UpperSaturationLimit=1  LowerSaturationLimit=-1  LinearizeAsGain=on  AntiWindupMode=clamping  Kb=1  LimitIntegrator=off  UpperIntegratorSaturationLimit=inf  LowerIntegratorSaturationLimit=-inf  POutMin=[]  POutMax=[]  IOutMin=[]  IOutMax=[]  DOutMin=[]  DOutMax=[]  NOutMin=[]  NOutMax=[]  SumOutMin=[]  SumOutMax=[]  SaturationOutMin=[]  SaturationOutMax=[]  PParamMin=[]  PParamMax=[]  IParamMin=[]  IParamMax=[]  DParamMin=[]  DParamMax=[]  NParamMin=[]  NParamMax=[]  KbParamMin=[]  KbParamMax=[]  KtParamMin=[]  KtParamMax=[]  KbOutMin=[]  KbOutMax=[]  KtOutMin=[]  KtOutMax=[]  IntegratorOutMin=[]  IntegratorOutMax=[]  FilterOutMin=[]  FilterOutMax=[]  SumI1OutMin=[]  SumI1OutMax=[]  SumI2OutMin=[]  SumI2OutMax=[]  SumI3OutMin=[]  SumI3OutMax=[]  SumI4OutMin=[]  SumI4OutMax=[]  SumDOutMin=[]  SumDOutMax=[]  DifferentiatorOutMin=[]  DifferentiatorOutMax=[]  FilterDiffOutCoefMin=[]  FilterDiffOutCoefMax=[]  ReciprocalOutMin=[]  ReciprocalOutMax=[]  SumDenOutMin=[]  SumDenOutMax=[]  SumNumOutMin=[]  SumNumOutMax=[]  DivideOutMin=[]  DivideOutMax=[]  UdiffTsProdOutMin=[]  UdiffTsProdOutMax=[]  NTsProdOutMin=[]  NTsProdOutMax=[]  UintegralTsProdOutMin=[]  UintegralTsProdOutMax=[]  UngainTsProdOutMin=[]  UngainTsProdOutMax=[]  ClampingZeroOutDataTypeStr=Inherit: Inherit via back propagation  ClampingZeroOutMin=[]  ClampingZeroOutMax=[]  FilterDenConstantOutDataTypeStr=Inherit: Inherit via back propagation  FilterDenConstantOutMin=[]  FilterDenConstantOutMax=[]  PCopyOutDataTypeStr=Inherit: Inherit via back propagation  PCopyOutMin=[]  PCopyOutMax=[]  NCopyOutDataTypeStr=Inherit: Inherit via back propagation  NCopyOutMin=[]  NCopyOutMax=[]  IntegratorContinuousStateAttributes=''  IntegratorStateMustResolveToSignalObject=off  IntegratorRTWStateStorageClass=Auto  FilterContinuousStateAttributes=''  FilterStateMustResolveToSignalObject=off  FilterRTWStateStorageClass=Auto  ParallelPVariant=InternalParameters  IdealPVariant=Disabled  IVariant=InternalParameters  DVariant=Disabled  IntegratorVariant=Continuous  SatVariant=Enabled  AWVariant=ContClampingParallel  PCopyVariant=Disabled  TRVariant=Disabled  FdbkBlocksVariant=Forward  IdealPFdbkVariant=Disabled  SatFdbkVariant=Disabled  DerivativeFilterVariant=Disabled  NVariant=Disabled  NCopyVariant=Disabled_SignalSpec  FilterICVariant=Disabled  IntegratorICVariant=InternalICs  ExternalResetVariant=Disabled  TRSumVariant=Passthrough  SumFdbkVariant=Disabled  SumVariant=Sum_PI  TsampFilterVariant=InternalTs  TsampNgainVariant=Passthrough  TsampIntegralVariant=Disabled_SignalSpec  ExternalSaturationOutDataTypeStr=Inherit: Same as second input  DerivativeSourceVariant=Disabled  PreIntVariant=InternalPreInt
  Pi exc. V ou Q : slpidlib/PID Controller  Controller=PI  Form=Parallel  TimeDomain=Continuous-time  UseExternalTs=off  SampleTime=-1  IntegratorMethod=Forward Euler  FilterMethod=Forward Euler  ControllerParametersSource=internal  P=5  I=5  UseKiTs=off  D=0  UseExternalDerivativeSource=off  N=100  UseFilter=on  TunerSelectOption=Transfer Function Based (PID Tuner App)  InitialConditionSource=internal  InitialConditionForIntegrator=0.5  InitialConditionForFilter=0  DifferentiatorICPrevScaledInput=0  ExternalReset=none  TrackingMode=off  Kt=1  LimitOutput=on  SatLimitsSource=internal  UpperSaturationLimit=10  LowerSaturationLimit=-10  LinearizeAsGain=on  AntiWindupMode=clamping  Kb=1  LimitIntegrator=off  UpperIntegratorSaturationLimit=inf  LowerIntegratorSaturationLimit=-inf  POutMin=[]  POutMax=[]  IOutMin=[]  IOutMax=[]  DOutMin=[]  DOutMax=[]  NOutMin=[]  NOutMax=[]  SumOutMin=[]  SumOutMax=[]  SaturationOutMin=[]  SaturationOutMax=[]  PParamMin=[]  PParamMax=[]  IParamMin=[]  IParamMax=[]  DParamMin=[]  DParamMax=[]  NParamMin=[]  NParamMax=[]  KbParamMin=[]  KbParamMax=[]  KtParamMin=[]  KtParamMax=[]  KbOutMin=[]  KbOutMax=[]  KtOutMin=[]  KtOutMax=[]  IntegratorOutMin=[]  IntegratorOutMax=[]  FilterOutMin=[]  FilterOutMax=[]  SumI1OutMin=[]  SumI1OutMax=[]  SumI2OutMin=[]  SumI2OutMax=[]  SumI3OutMin=[]  SumI3OutMax=[]  SumI4OutMin=[]  SumI4OutMax=[]  SumDOutMin=[]  SumDOutMax=[]  DifferentiatorOutMin=[]  DifferentiatorOutMax=[]  FilterDiffOutCoefMin=[]  FilterDiffOutCoefMax=[]  ReciprocalOutMin=[]  ReciprocalOutMax=[]  SumDenOutMin=[]  SumDenOutMax=[]  SumNumOutMin=[]  SumNumOutMax=[]  DivideOutMin=[]  DivideOutMax=[]  UdiffTsProdOutMin=[]  UdiffTsProdOutMax=[]  NTsProdOutMin=[]  NTsProdOutMax=[]  UintegralTsProdOutMin=[]  UintegralTsProdOutMax=[]  UngainTsProdOutMin=[]  UngainTsProdOutMax=[]  ClampingZeroOutDataTypeStr=Inherit: Inherit via back propagation  ClampingZeroOutMin=[]  ClampingZeroOutMax=[]  FilterDenConstantOutDataTypeStr=Inherit: Inherit via back propagation  FilterDenConstantOutMin=[]  FilterDenConstantOutMax=[]  PCopyOutDataTypeStr=Inherit: Inherit via back propagation  PCopyOutMin=[]  PCopyOutMax=[]  NCopyOutDataTypeStr=Inherit: Inherit via back propagation  NCopyOutMin=[]  NCopyOutMax=[]  IntegratorContinuousStateAttributes=''  IntegratorStateMustResolveToSignalObject=off  IntegratorRTWStateStorageClass=Auto  FilterContinuousStateAttributes=''  FilterStateMustResolveToSignalObject=off  FilterRTWStateStorageClass=Auto  ParallelPVariant=InternalParameters  IdealPVariant=Disabled  IVariant=InternalParameters  DVariant=Disabled  IntegratorVariant=Continuous  SatVariant=Enabled  AWVariant=ContClampingParallel  PCopyVariant=Disabled  TRVariant=Disabled  FdbkBlocksVariant=Forward  IdealPFdbkVariant=Disabled  SatFdbkVariant=Disabled  DerivativeFilterVariant=Disabled  NVariant=Disabled  NCopyVariant=Disabled_SignalSpec  FilterICVariant=Disabled  IntegratorICVariant=InternalICs  ExternalResetVariant=Disabled  TRSumVariant=Passthrough  SumFdbkVariant=Disabled  SumVariant=Sum_PI  TsampFilterVariant=InternalTs  TsampNgainVariant=Passthrough  TsampIntegralVariant=Disabled_SignalSpec  ExternalSaturationOutDataTypeStr=Inherit: Same as second input  DerivativeSourceVariant=Disabled  PreIntVariant=InternalPreInt
  Subtract : Sum  Inputs=+-
  Subtract1 : Sum  Inputs=+-
  Subtract2 : Sum  Inputs=|+-
  Subtract6 : Sum  Inputs=|+-
  Transfer Fcn : TransferFcn  Denominator=[1e-4 10]
  Transfer Fcn1 : TransferFcn  Denominator=[0.01 100]
  Transport Delay : TransportDelay  DelayTime=0.01
  Transport Delay1 : TransportDelay  DelayTime=0.001
  V0 : Bias  Bias=265.6  SaturateOnIntegerOverflow=off
  Vref : Constant  Value=220
  f0 : Bias  Bias=65  SaturateOnIntegerOverflow=off
  p/(2*pi) : Gain  Gain=1/pi
  Acelerador : Outport
  Excitação : Outport  Port=2
  wires:
  w (rad/s)/1 -> p/(2*pi)/1
  Dynamic RMS/1 -> Transport Delay1/1  "VGS_rms"
  VGS/1 -> Dynamic RMS/1
  Fe (Hz)/1 -> Subtract6/1
  p/(2*pi)/1 -> Transport Delay/1  "fe"
  Subtract6/1 -> PI acel. Freq ou Potencia Ativa/1
  Subtract2/1 -> Pi exc. V ou Q/1
  Vref/1 -> Subtract2/1
  Pi exc. V ou Q/1 -> V0/1
  Subtract1/1 -> Transfer Fcn1/1
  Transport Delay/1 -> Subtract6/2, Subtract/2  "fe"
  Subtract/1 -> Transfer Fcn/1
  Transfer Fcn/1 -> Acelerador/1
  f0/1 -> Subtract/1  "f0"
  Transfer Fcn1/1 -> Excitação em V0/1
  Transport Delay1/1 -> Subtract1/2, Subtract2/2  "VGS_rms"
  V0/1 -> Subtract1/1  "v0"
  Excitação em V0/1 -> Excitação/1
  PI acel. Freq ou Potencia Ativa/1 -> f0/1

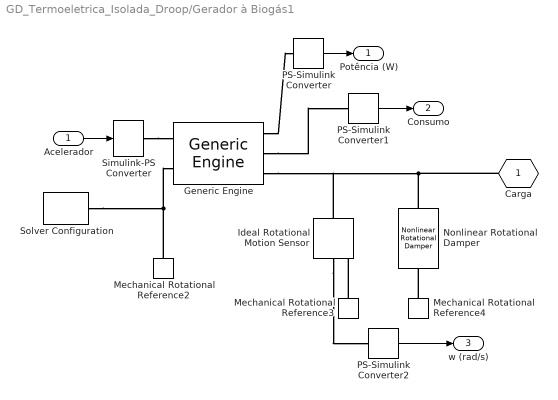
== system GD_Termoeletrica_Isolada_Droop/Gerador à Biogás1 ==
  Acelerador : Inport
  Generic Engine : sdl_lib/Engines & Motors/Generic Engine  input_type=sdl.enum.GenericEngineInputType.NormalizedThrottle  model_parameterization=1  engine_type=1  Trq_max=380 N*m  w_Trq_max=4300 rpm  P_max=20 kW  w_P_max=4.5e+3 rpm  w_max=6e+3 rpm  w_min=200 rpm  w_tab=[ 500 1000 2e+3 3e+3 4e+3 5e+3 6e+3 7e+3 ] rpm  trq_tab=[ 380 380 380 380 350 280 200 80 ] N*m  pwr_tab=[ 2e+4 4e+4 7.8e+4 1.2e+5 1.45e+5 1.48e+5 1.25e+5 6e+4 ] W  interp_method=1  w_thr=5000 rpm  model_inertia=1  inertia=0.01 kg*m^2  initial_velocity=500 rpm  model_time_constant=0  time_constant=0.2 s  initial_normalized_throttle=0  fc_model=1  fc_per_rev=25 mg/rev  fc_w_tab=[ 1000 2e+3 3e+3 4e+3 5e+3 6e+3 ] rpm  fc_trq_tab=[ 0 80 160 200 240 320 360 400 ] N*m  fc_tab=[ 0.5 0.9 1.4 1.6 1.9 2.7 3.4 4.4; 1 1.7 2.7 3.1 3.6 5 6 7.4; 1.4 2.7 4 4.8 5.6 7.5 8.5 10.5; 2 3.6 5.8 6.7 8 10.4 11.7 13.3; 2.5 4.8 7.9 9.4 10.8 14 16.2 18.6; 3.1 6 10.3 11.9 13.8 18.4 22 26.5 ] g/s  bmep_tab=[ 0 250 500 625 750 1000 1.15e+3 1.25e+3 ] kPa  bsfc_tab=[ 410 380 300 280 270 290 320 380; 410 370 290 270 260 270 285 320; 415 380 290 275 265 270 270 300; 420 390 310 290 285 280 280 285; 430 410 340 320 310 300 310 320; 450 430 370 340 330 330 350 380 ] g/hr/kW  fc_interp_method=1  displaced_volume=400 cm^3  rev_per_cycle=2  idle_speed=0  idle_speed_reference=1000 rpm  tau_controller=1 s  idle_w_thr=1 rpm  redline=false  redline_speed=5000 rpm  tau_redline=1 s  redline_w_thr=1 rpm
      settings: InternalSimscapePortConfiguration="{\"Bottom\":[],\"Left\":[{\"id\":\"ThrNorm\",\"label\":\"Thr\",\"type\":\"input\"},{\"id\":\"B\",\"label\":\"B\",\"type\":\"foundation.mechanical.rotational.rotational\"}],\"Right\":[{\"id\":\"P\",\"label\":\"P\",\"type\":\"output\"},{\"id\":\"FC\",\"label\":\"FC\",\"type\":\"output\"},{\"id\":\"F\",\"label\":\"F\",\"type\":\"foundation.mechanical.rotational.rotational\"}],\"Top\":[]}"
  Ideal Rotational Motion Sensor : fl_lib/Mechanical/Mechanical Sensors/Ideal Rotational Motion Sensor  reference=foundation.enum.MeasurementReference.difference  acceleration_port=false  velocity_port=true  position_port=true  wrap_angle=false  offset=0 rad
  Mechanical Rotational Reference2 : fl_lib/Mechanical/Rotational Elements/Mechanical Rotational Reference
  Mechanical Rotational Reference3 : fl_lib/Mechanical/Rotational Elements/Mechanical Rotational Reference
  Mechanical Rotational Reference4 : fl_lib/Mechanical/Rotational Elements/Mechanical Rotational Reference
  Nonlinear Rotational Damper : sdl_lib/Couplings & Drives/Springs & Dampers/Nonlinear Rotational Damper  parameterization=1  symmetry=1  coefficient_vector=[1e-6 0 1e-7 0 0] N*m/(rad/s)  positive_coefficient_vector=[ 1e-4 0 1e-5 0 1e-6 ] N*m/(rad/s)  negative_coefficient_vector=[ 0.001 -1e-5 1e-4 0 0 ] N*m/(rad/s)  angular_velocity_vector=[ -1 -0.5 -0.3 -0.1 0.1 0.3 0.5 1 ] rad/s  torque_vector=[ -0.001 -4e-4 -2e-4 -5e-5 5e-5 2e-4 4e-4 0.001 ] N*m  interp_method=1  extrap_method=1
      settings: InternalSimscapePortConfiguration="{\"Bottom\":[],\"Left\":[{\"id\":\"R\",\"label\":\"R\",\"type\":\"foundation.mechanical.rotational.rotational\"}],\"Right\":[{\"id\":\"C\",\"label\":\"C\",\"type\":\"foundation.mechanical.rotational.rotational\"}],\"Top\":[]}"
  PS-Simulink Converter : nesl_utility/PS-Simulink Converter  PhysicalDomain=network_engine_domain  SubClassName=ps_output  LeftPortType=input  RightPortType=output  PseudoPeriodic=off  Frequencies=[]  VectorFormat=1-D array  Unit=1  AffineConversion=off
  PS-Simulink Converter1 : nesl_utility/PS-Simulink Converter  PhysicalDomain=network_engine_domain  SubClassName=ps_output  LeftPortType=input  RightPortType=output  PseudoPeriodic=off  Frequencies=[]  VectorFormat=1-D array  Unit=1  AffineConversion=off
  PS-Simulink Converter2 : nesl_utility/PS-Simulink Converter  PhysicalDomain=network_engine_domain  SubClassName=ps_output  LeftPortType=input  RightPortType=output  PseudoPeriodic=off  Frequencies=[]  VectorFormat=1-D array  Unit=1  AffineConversion=off
  Simulink-PS Converter : nesl_utility/Simulink-PS Converter  PhysicalDomain=network_engine_domain  SubClassName=ps_input  LeftPortType=input  RightPortType=output  PseudoPeriodic=off  Frequencies=[]  NoiseDistribution=none  NoiseParameters=[]  Unit=1  AffineConversion=off  FilteringAndDerivatives=zero  SimscapeFilterOrder=1  InputFilterTimeConstant=0.001  UdotUserProvided=1
  Solver Configuration : nesl_utility/Solver Configuration  PhysicalDomain=network_engine_domain  SubClassName=solver  LeftPortType=input  RightPortType=generic  Tones=[]  Harmonics=[]  SimulateNoise=off  Profile=off  UseLocalSampling=off  EnableSwitchedLinearOptims=on  FrequencyDomain=off  UseCCode=off  RelTol=0.001  AbsTol=1e-06  MinStep=1e-09  ToWorkspace=off  RevertToSquareIcSolve=off  NumHomotopyIterations=100  PhasorMode=off  PhasorModeNumHarmonics=1  ConsistencySolver=NEWTON_FTOL  IndexReductionMethod=DerivativeReplacement  DoDC=off  ResidualTolerance=1e-09  ConsistencyTolSource=GLOBAL  ConsistencyAbsTol=0.001  ConsistencyRelTol=0.001  ConsistencyTolFactor=0.001  UseLocalSolver=on  LocalSolverChoice=NE_BACKWARD_EULER_ADVANCER  ResolveIndetEquations=on  FunctionEvalNumThread=1  LocalSolverSampleTime=0.0001  DoFixedCost=on  MaxNonlinIter=4  MaxModeIter=2  ComputeImpulses=off  ImpulseIterations=2  LinearAlgebra=Sparse  LinearAlgebraNumThread=0  EquationFormulation=NE_TIME_EF  DelaysMemoryBudget=1024  AutomaticFiltering=on  FilteringTimeConstant=0.001  PartitionStorageMethod=AS_NEEDED  PartitionMemoryBudget=1024  PartitionMethod=FAST  MultibodyUseLocalSolver=off  MultibodyLocalSolverChoice=ODE1  MultibodyLocalSolverSampleTime=0.001
  Carga : PMIOPort  Tag=PMCPort  Side=Right
  Potência (W) : Outport
  Consumo : Outport  Port=2
  w (rad/s) : Outport  Port=3
  wires:
  Acelerador/1 -> Simulink-PS Converter/1
  PS-Simulink Converter/1 -> Potência (W)/1
  PS-Simulink Converter1/1 -> Consumo/1
  PS-Simulink Converter2/1 -> w (rad/s)/1
  connections:
  Solver Configuration/RConn1 -- Mechanical Rotational Reference2/LConn1 -- Generic Engine/LConn2
  Generic Engine/RConn1 -- PS-Simulink Converter/LConn1
  Simulink-PS Converter/RConn1 -- Generic Engine/LConn1
  Generic Engine/RConn2 -- PS-Simulink Converter1/LConn1
  Ideal Rotational Motion Sensor/LConn1 -- Generic Engine/RConn3 -- Carga/RConn1 -- Nonlinear Rotational Damper/LConn1
  Ideal Rotational Motion Sensor/RConn2 -- PS-Simulink Converter2/LConn1
  Mechanical Rotational Reference3/LConn1 -- Ideal Rotational Motion Sensor/RConn1
  Mechanical Rotational Reference4/LConn1 -- Nonlinear Rotational Damper/RConn1

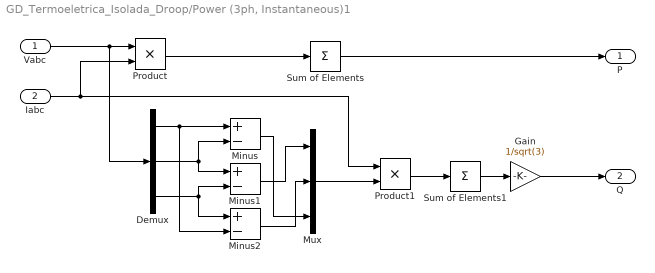
== system GD_Termoeletrica_Isolada_Droop/Power (3ph, Instantaneous)1 ==
  Vabc : Inport
  Iabc : Inport  Port=2
  Demux : Demux  Outputs=3
  Gain : Gain  Gain=1/sqrt(3)
  Minus : Sum  Inputs=+-
  Minus1 : Sum  Inputs=+-
  Minus2 : Sum  Inputs=+-
  Mux : Mux  Inputs=3
  Product : Product
  Product1 : Product
  Sum of Elements : Sum  Inputs=+
  Sum of Elements1 : Sum  Inputs=+
  P : Outport  VectorParamsAs1DForOutWhenUnconnected=off
  Q : Outport  Port=2  VectorParamsAs1DForOutWhenUnconnected=off
  wires:
  Minus/1 -> Mux/3
  Minus2/1 -> Mux/2
  Minus1/1 -> Mux/1
  Gain/1 -> Q/1
  Sum of Elements1/1 -> Gain/1
  Product1/1 -> Sum of Elements1/1
  Mux/1 -> Product1/2
  Demux/3 -> Minus1/2, Minus2/1
  Demux/2 -> Minus/2, Minus1/1
  Demux/1 -> Minus/1, Minus2/2
  Sum of Elements/1 -> P/1
  Product/1 -> Sum of Elements/1
  Iabc/1 -> Product/2, Product1/1
  Vabc/1 -> Product/1, Demux/1
